simulink model "LDR"  (R2023b)
settings: Solver=FixedStepDiscrete  StartTime=0.0  StopTime=10.0  FixedStep=0.01  RelTol=1e-3
settings Model: Creator=LENOVO-MCC  LastModifiedBy=LENOVO-MCC
settings OptimizationCC: DefaultParameterBehavior=Inlined  EnhancedBackFolding=on  PassReuseOutputArgsAs=Individual arguments  ZeroExternalMemoryAtStartup=off  ZeroInternalMemoryAtStartup=off  OptimizeBlockOrder=speed  DifferentSizesBufferReuse=on  OptimizationCustomize=off  EfficientTunableParamExpr=on
settings DebuggingCC: ParameterTunabilityLossMsg=error
settings SFSimCC: MATLABDynamicMemAlloc=off
settings RTWCC: Description=Embedded Coder  SystemTargetFile=ert.tlc  GenCodeOnly=on  TemplateMakefile=ert_default_tmf  GenerateReport=on  LaunchReport=on  GenerateCodeMetricsReport=on
settings CodeAppCC: ForceParamTrailComments=on  IgnoreCustomStorageClasses=off  OperatorAnnotations=on  SimulinkDataObjDesc=on  SFDataObjDesc=on  InsertBlockDesc=on
settings ERTTargetCC: TargetLangStandard=C99 (ISO)  GenerateSampleERTMain=on  InlinedParameterPlacement=NonHierarchical  ERTCustomFileTemplate=example_file_process.tlc

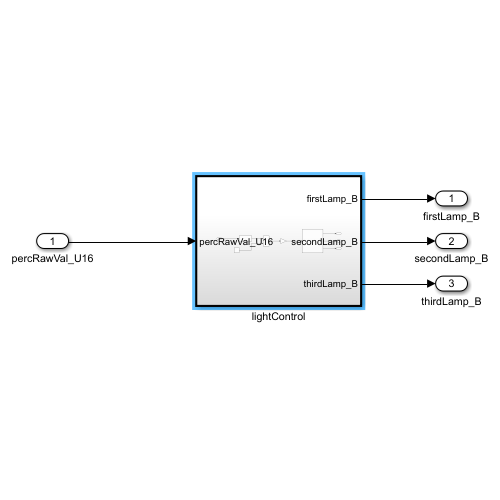
[thumbnail: Simulink's stored preview of the top-level diagram]
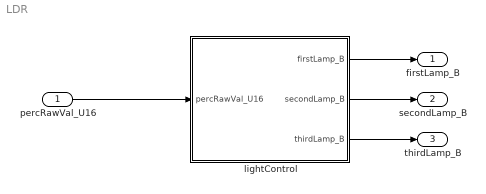
== system LDR ==
  percRawVal_U16 : Inport  OutDataTypeStr=uint16
  lightControl : Subsystem  TreatAsAtomicUnit=on
      settings: RTWFcnNameOpts=Use subsystem name  RTWFileNameOpts=Use subsystem name
  firstLamp_B : Outport  OutDataTypeStr=boolean
  secondLamp_B : Outport  Port=2  OutDataTypeStr=boolean
  thirdLamp_B : Outport  Port=3  OutDataTypeStr=boolean
  wires:
  percRawVal_U16/1 -> lightControl/1(percRawVal_U16)
  lightControl/1(firstLamp_B) -> firstLamp_B/1
  lightControl/2(secondLamp_B) -> secondLamp_B/1
  lightControl/3(thirdLamp_B) -> thirdLamp_B/1

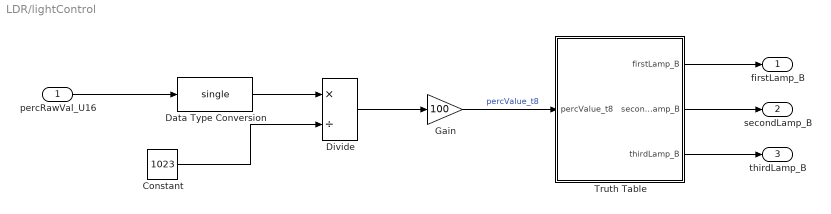
== system LDR/lightControl ==
  percRawVal_U16 : Inport  OutDataTypeStr=uint16
  Constant : Constant  Value=1023  OutDataTypeStr=single
  Data Type Conversion : DataTypeConversion  OutDataTypeStr=single  SaturateOnIntegerOverflow=off  RndMeth=Floor
  Divide : Product  Inputs=*/
  Gain : Gain  Gain=100  OutDataTypeStr=int8
  Truth Table : Truth Table  TreatAsAtomicUnit=on
  firstLamp_B : Outport  OutDataTypeStr=boolean
  secondLamp_B : Outport  Port=2  OutDataTypeStr=boolean
  thirdLamp_B : Outport  Port=3  OutDataTypeStr=boolean
  wires:
  percRawVal_U16/1 -> Data Type Conversion/1
  Data Type Conversion/1 -> Divide/1
  Constant/1 -> Divide/2
  Divide/1 -> Gain/1
  Gain/1 -> Truth Table/1(percValue_t8)  "percValue_t8"
  Truth Table/1(firstLamp_B) -> firstLamp_B/1
  Truth Table/2(secondLamp_B) -> secondLamp_B/1
  Truth Table/3(thirdLamp_B) -> thirdLamp_B/1

== matlab function LDR/lightControl/Truth Table ==
  data: percValue_t8 input; firstLamp_B output boolean; secondLamp_B output boolean; thirdLamp_B output boolean
function [firstLamp_B, secondLamp_B, thirdLamp_B] = fcn(percValue_t8)

aVarTruthTableCondition_1 = false;
aVarTruthTableCondition_2 = false;
aVarTruthTableCondition_3 = false;


% Example condition 1

aVarTruthTableCondition_1 = logical(percValue_t8 > 60);

% Example condition 2

aVarTruthTableCondition_2 = logical(percValue_t8 > 40);

% Condition #3
aVarTruthTableCondition_3 = logical(percValue_t8 > 20);

if (aVarTruthTableCondition_1)
    aFcnTruthTableAction_1();
elseif (aVarTruthTableCondition_2)
    aFcnTruthTableAction_2();
elseif (aVarTruthTableCondition_3)
    aFcnTruthTableAction_3();
else % Default
    aFcnTruthTableAction_4();
end

function aFcnTruthTableAction_1()

% Example action 1 called from D1 & D2 column in condition table

firstLamp_B =true;
secondLamp_B =true;
thirdLamp_B =true;

function aFcnTruthTableAction_2()

% Example action 2 called from D3 column in condition table

firstLamp_B =true;
secondLamp_B =true;
thirdLamp_B =false;

function aFcnTruthTableAction_3()



firstLamp_B =true;
secondLamp_B =false;
thirdLamp_B =false;

function aFcnTruthTableAction_4()



firstLamp_B =false;
secondLamp_B =false;
thirdLamp_B =false;
